simulink model "least_square_2ordem_p3"  (R2024b)
settings: Solver=ode45  StartTime=10  StopTime=20  RelTol=1e-3  AbsTol=1e-6
values from neighbouring files (symbols this model uses):
  Aq = 2    [sim_grad_norm_2ordem.m]
  As = 2    [sim_grad_norm.m]    (also in sim_grad_norm_2ordem.m = 0)
  DC = 1    [sim_grad_norm.m]    (also in sim_grad_norm_2ordem.m)
  kappa = 0    [sim_grad_norm.m]    (also in sim_grad_norm_2ordem.m = 1)
  lambda0 = 1    [sim_grad_norm.m]    (also in sim_grad_norm_2ordem.m)
  lambda1 = 2    [sim_grad_norm.m]    (also in sim_grad_norm_2ordem.m)
  P0 = 1*eye(4)    [sim_grad_norm.m]    (also in sim_grad_norm_2ordem.m)
  st = 0.01    [sim_grad_norm.m]    (also in sim_grad_norm_2ordem.m)
  theta0 = [0;0;0;0]    [sim_grad_norm.m]    (also in sim_grad_norm_2ordem.m)
  theta_star2 = [b0; b1; a0; a1]    [sim_grad_norm.m]    (also in sim_grad_norm_2ordem.m)
  wq = 0.1*pi    (= 0.314159265359)    [sim_grad_norm_2ordem.m]
  ws = 0.1*pi    (= 0.314159265359)    [sim_grad_norm.m]    (also in sim_grad_norm_2ordem.m = 3.14159265359)
libraries: cstblocks x1
settings Model: Creator=Ramon  LastModifiedBy=sarin
settings SolverCC: AutoScaleAbsTol=off  AlgebraicLoopSolver=TrustRegion
settings DataIOCC: SaveFormat=Array  SignalLoggingSaveFormat=ModelDataLogs  SaveOutput=off  SaveTime=off  ReturnWorkspaceOutputs=off
settings OptimizationCC: BlockReduction=off  BooleanDataType=off  ExpressionDepthLimit=2147483647  InitFltsAndDblsToZero=on  LifeSpan=inf
settings DebuggingCC: SaveWithParameterizedLinksMsg=none  UnderspecifiedInitializationDetection=Classic  MergeDetectMultiDrivingBlocksExec=none  SignalResolutionControl=TryResolveAllWithWarning  MultiTaskDSMMsg=warning  MultiTaskCondExecSysMsg=none  FcnCallInpInsideContextMsg=warning  UnconnectedInputMsg=warning  UnconnectedOutputMsg=warning  UnconnectedLineMsg=warning  StateNameClashWarn=warning  SFUnexpectedBacktrackingDiag=warning  SFNoUnconditionalDefaultTransitionDiag=warning  SFExecutionAtInitializationDiag=none  ArithmeticOperatorsInVariantConditions=warning
settings HardwareCC: ProdBitPerPointer=32  ProdBitPerSizeT=32  ProdBitPerPtrDiffT=32  ProdLargestAtomicFloat=None  ProdIntDivRoundTo=Undefined  ProdEndianess=Unspecified  ProdWordSize=32  ProdHWDeviceType=32-bit Generic  TargetUnknown=on
settings ModelReferenceCC: EnableRefExpFcnMdlSchedulingChecks=on  PropagateSignalLabelsOutOfModel=off
settings SFSimCC: SimUseLocalCustomCode=off  CustomCodeUndefinedFunction=UseInterfaceOnly
settings RTWCC: TemplateMakefile=grt_vc.tmf  RTWUseLocalCustomCode=off  GPUComputeCapability=3.5  DLArmComputeVersion=19.05
settings CodeAppCC: StateflowObjectComments=on
settings GRTTargetCC: TargetLangStandard=C89/C90 (ANSI)  CombineOutputUpdateFcns=off  GRTInterface=on
settings ConfigComp: CovMetricSettings=dw  CovSaveCumulativeToWorkspaceVar=on  CovSaveSingleToWorkspaceVar=on  CovExternalEMLEnable=off

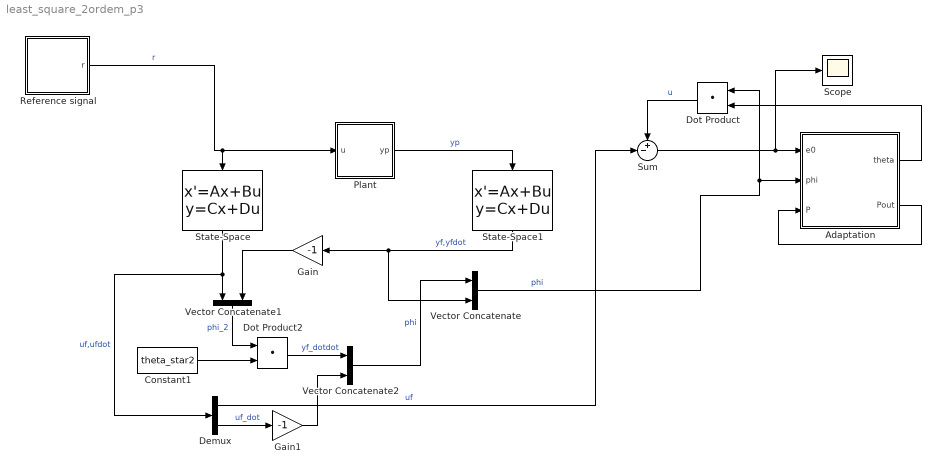
== system least_square_2ordem_p3 ==
  Adaptation : Subsystem
  Constant1 : Constant  Value=theta_star2
  Demux : Demux  Outputs=2
  Dot Product : DotProduct  OutDataTypeStr=Inherit: Inherit via internal rule
  Dot Product2 : DotProduct  OutDataTypeStr=Inherit: Inherit via internal rule
  Gain : Gain  Gain=-1
  Gain1 : Gain  Gain=-1
  Plant : Subsystem
  Reference signal : Subsystem
  Scope : Scope
  State-Space : StateSpace  A=[0 1; -lambda0 -lambda1]  B=[0; 1]  C=[1 0;0 1]  D=[0; 0]  InitialCondition=0
  State-Space1 : StateSpace  A=[0 1; -lambda0 -lambda1]  B=[0; 1]  C=[1 0;0 1]  D=[0; 0]  InitialCondition=0
  Sum : Sum  Inputs=+-|
  Vector Concatenate : Concatenate
  Vector Concatenate1 : Concatenate
  Vector Concatenate2 : Concatenate
  wires:
  Adaptation/1(theta) -> Dot Product/2
  Vector Concatenate/1 -> Adaptation/2(phi), Dot Product/1  "phi"
  Reference signal/1(r) -> State-Space/1, Plant/1(u)  "r"
  Plant/1(yp) -> State-Space1/1  "yp"
  State-Space1/1 -> Vector Concatenate/2, Gain/1  "yf,yfdot"
  State-Space/1 -> Vector Concatenate1/1, Demux/1  "uf,ufdot"
  Sum/1 -> Adaptation/1(e0), Scope/1
  Dot Product/1 -> Sum/1  "u"
  Gain/1 -> Vector Concatenate1/2
  Vector Concatenate1/1 -> Dot Product2/1  "phi_2"
  Constant1/1 -> Dot Product2/2
  Dot Product2/1 -> Vector Concatenate2/1  "yf_dotdot"
  Demux/2 -> Gain1/1  "uf_dot"
  Gain1/1 -> Vector Concatenate2/2
  Vector Concatenate2/1 -> Vector Concatenate/1  "phi"
  Demux/1 -> Sum/2  "uf"
  Adaptation/2(Pout) -> Adaptation/3(P)

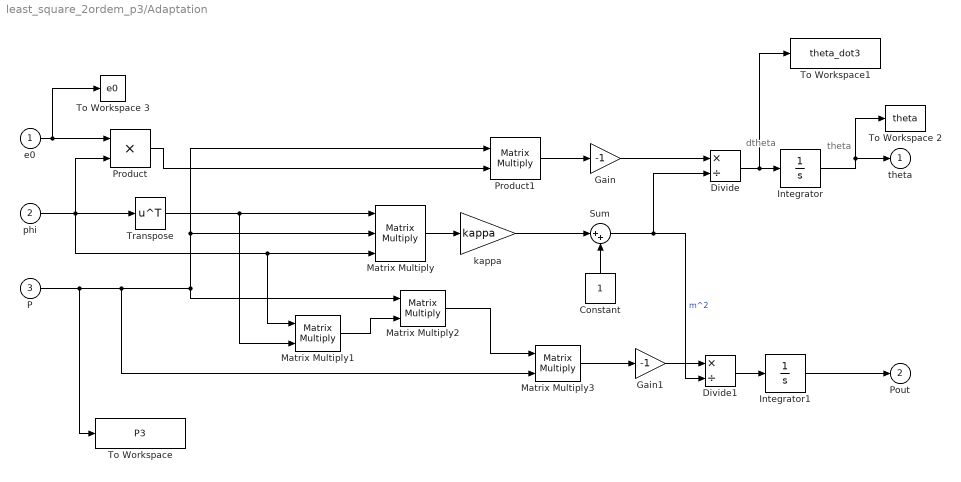
== system least_square_2ordem_p3/Adaptation ==
  note: dtheta
  note: theta
  e0 : Inport  PortDimensions=1
  phi : Inport  Port=2
  P : Inport  Port=3
  Constant : Constant
  Divide : Product  Inputs=*/
  Divide1 : Product  Inputs=*/
  Gain : Gain  Gain=-1
  Gain1 : Gain  Gain=-1
  Integrator : Integrator  InitialCondition=theta0
  Integrator1 : Integrator  InitialCondition=P0
  Matrix Multiply : Product  Inputs=3  Multiplication=Matrix(*)
  Matrix Multiply1 : Product  Multiplication=Matrix(*)
  Matrix Multiply2 : Product  Multiplication=Matrix(*)
  Matrix Multiply3 : Product  Multiplication=Matrix(*)
  Product : Product  InputSameDT=on  RndMeth=Zero  SaturateOnIntegerOverflow=on  OutDataTypeStr=Inherit: Same as first input
  Product1 : Product  Multiplication=Matrix(*)
  Sum : Sum  Inputs=|++
  To Workspace : ToWorkspace  VariableName=P3  SaveFormat=Structure With Time  SampleTime=-1
  To Workspace 2 : ToWorkspace  VariableName=theta  SampleTime=st
  To Workspace 3 : ToWorkspace  VariableName=e0  SampleTime=st
  To Workspace1 : ToWorkspace  VariableName=theta_dot3  SaveFormat=Structure With Time  SampleTime=-1
  Transpose : Math  Operator=transpose
  kappa : Gain  Gain=kappa  SaturateOnIntegerOverflow=on  OutDataTypeStr=Inherit: Same as input  ParamDataTypeStr=Inherit: Same as input
  theta : Outport  InitialOutput=0  VectorParamsAs1DForOutWhenUnconnected=off
  Pout : Outport  Port=2  InitialOutput=0  VectorParamsAs1DForOutWhenUnconnected=off
  wires:
  Divide1/1 -> Integrator1/1
  Matrix Multiply/1 -> kappa/1
  Matrix Multiply2/1 -> Matrix Multiply3/1
  Gain1/1 -> Divide1/1
  Matrix Multiply1/1 -> Matrix Multiply2/2
  Divide/1 -> To Workspace1/1, Integrator/1
  Product/1 -> Product1/2
  Constant/1 -> Sum/2
  Gain/1 -> Divide/1
  Integrator/1 -> To Workspace 2/1, theta/1
  Sum/1 -> Divide1/2, Divide/2  "m^2"
  Transpose/1 -> Matrix Multiply1/2, Matrix Multiply/1
  P/1 -> To Workspace/1, Matrix Multiply3/2, Matrix Multiply2/1, Matrix Multiply/2, Product1/1
  Integrator1/1 -> Pout/1
  Product1/1 -> Gain/1
  kappa/1 -> Sum/1
  phi/1 -> Transpose/1, Matrix Multiply1/1, Matrix Multiply/3, Product/2
  e0/1 -> Product/1, To Workspace 3/1
  Matrix Multiply3/1 -> Gain1/1

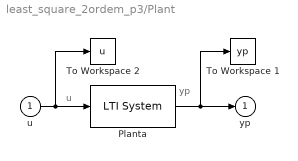
== system least_square_2ordem_p3/Plant ==
  note: yp
  note: u
  u : Inport
  Planta : cstblocks/LTI System  sys=P  IC=x0  PadeOrder=0
  To Workspace 1 : ToWorkspace  VariableName=yp  SampleTime=st
  To Workspace 2 : ToWorkspace  VariableName=u  SampleTime=st
  yp : Outport  InitialOutput=0  VectorParamsAs1DForOutWhenUnconnected=off
  wires:
  u/1 -> To Workspace 2/1, Planta/1
  Planta/1 -> yp/1, To Workspace 1/1

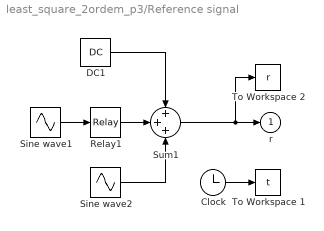
== system least_square_2ordem_p3/Reference signal ==
  Clock : Clock
  DC1 : Constant  Value=DC
  Relay1 : Relay  OnOutputValue=Aq  OffOutputValue=-Aq
  Sine wave1 : Sin  Frequency=wq  SampleTime=0
  Sine wave2 : Sin  Amplitude=As  Frequency=ws  SampleTime=0
  Sum1 : Sum  Inputs=+++  InputSameDT=on  SaturateOnIntegerOverflow=on  OutDataTypeStr=Inherit: Same as first input
  To Workspace 1 : ToWorkspace  VariableName=t  SampleTime=st
  To Workspace 2 : ToWorkspace  VariableName=r  SampleTime=st
  r : Outport  InitialOutput=0  VectorParamsAs1DForOutWhenUnconnected=off
  wires:
  Clock/1 -> To Workspace 1/1
  Sine wave2/1 -> Sum1/3
  Sum1/1 -> r/1, To Workspace 2/1
  DC1/1 -> Sum1/1
  Relay1/1 -> Sum1/2
  Sine wave1/1 -> Relay1/1
